simulink model "P4p3"  (R2014a)
settings: Solver=ode1  StartTime=0.0  StopTime=inf  FixedStep=0.002  RelTol=1e-3
PostLoadFcn:
  | qc_set_target_type(getConfigSet(bdroot, 'QUARC Default Target Configuration'));
undefined symbols (not defined in the file): A, B, C_elev_trav, HIL, Joystick_gain_x, Joystick_gain_y, K_P, L_elev_trav_real, P_P, qc_get_step_size, Vd_star, Vs_star
libraries: simulink_extras x6, quarc_library x4
settings Model: SimulationMode=external  ExtModeTrigDuration=15000  Creator=Rchan  LastModifiedBy=tikjetsa
settings SolverCC: PositivePriorityOrder=on
settings DataIOCC: SignalLoggingSaveFormat=ModelDataLogs
settings OptimizationCC: ExpressionDepthLimit=2147483647  InitFltsAndDblsToZero=on
settings DebuggingCC: SaveWithParameterizedLinksMsg=none  UnderspecifiedInitializationDetection=Classic  MultiTaskDSMMsg=warning  MultiTaskCondExecSysMsg=none  FcnCallInpInsideContextMsg=UseLocalSettings  StateNameClashWarn=warning
settings RTWCC: SystemTargetFile=quarc_win64.tlc  TemplateMakefile=quarc_default_tmf  Description=QUARC Win64 Target  ProcessScript=quarc_win64_make_rtw_hook
settings STFCustomTargetCC: CPPClassGenCompliant=on
settings GRTTargetCC: ParMdlRefBuildCompliant=off  CompOptLevelCompliant=off  CombineOutputUpdateFcns=off  MatFileLogging=off  GRTInterface=on  ExtMode=on  ExtModeMexFile=quarc_comm

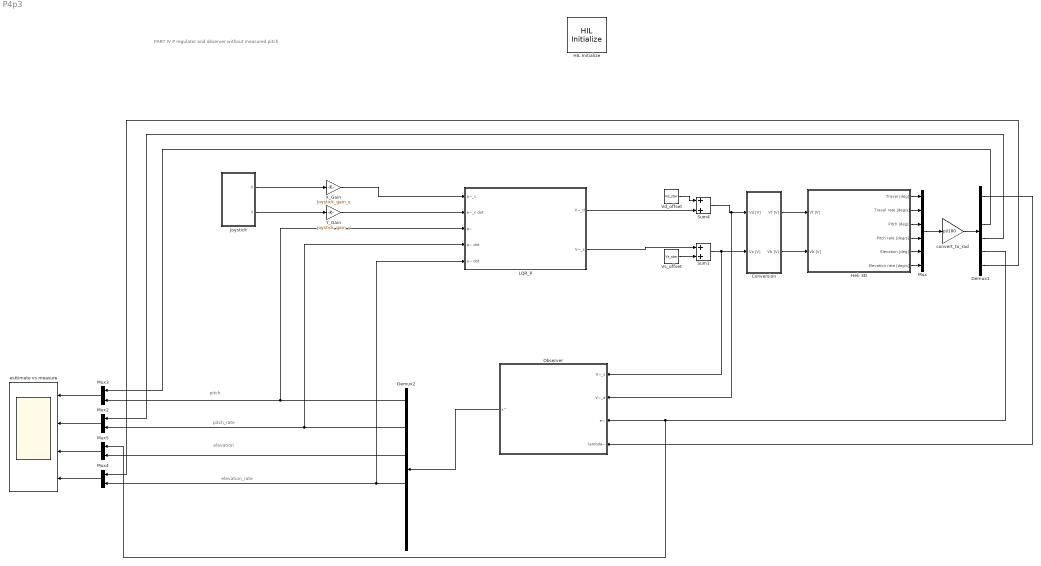
== system P4p3 ==
  note: elevation_rate
  note: elevation
  note: pitch_rate
  note: pitch
  note: PART IV
      | P regulator and observer without measured pitch
  Conversion : Subsystem
  Demux1 : Demux  Outputs=6
  Demux2 : Demux  Outputs=6
  HIL Initialize : quarc_library/Data Acquisition/Generic/Configuration/HIL Initialize  Priority=-99  object_name=HIL-1  board_type=q8_usb  board_number=0  board_options=update_rate=normal;decimation=1  exclusive=off  active=off  hardware_clocks=[0:2]  clock_modes=[]  initial_clock_frequencies=[]  set_clock_params_at_start=off  set_clock_params_at_switch_in=off  set_clock_frequencies_at_start=off  set_clock_frequencies_at_switch_in=off  analog_input_channels=[0:7]  analog_input_maximums=10  analog_input_minimums=-10  set_analog_input_params_at_start=on  set_analog_input_params_at_switch_in=off  analog_output_channels=[0:7]  analog_output_maximums=10  analog_output_minimums=-10  initial_analog_outputs=[0]  final_analog_outputs=[0]  watchdog_analog_outputs=0  set_analog_output_params_at_start=on  set_analog_output_params_at_switch_in=off  set_analog_outputs_at_start=on  set_analog_outputs_at_switch_in=off  set_analog_outputs_at_terminate=on  set_analog_outputs_at_switch_out=off  set_analog_outputs_on_watchdog=off  digital_input_channels=[]  digital_output_channels=[]  digital_output_configuration=[]  initial_digital_outputs=[1]  final_digital_outputs=[1]  watchdog_digital_outputs=[1]  set_digital_output_params_at_start=off  set_digital_output_params_at_switch_in=off  set_digital_outputs_at_start=on  set_digital_outputs_at_switch_in=off  set_digital_outputs_at_terminate=on  set_digital_outputs_at_switch_out=off  set_digital_outputs_on_watchdog=off  encoder_channels=[0:7]  quadrature=[4]  encoder_filter_frequency=[]  initial_encoder_counts=[0]  set_encoder_params_at_start=on  set_encoder_params_at_switch_in=off  set_encoder_counts_at_start=on  set_encoder_counts_at_switch_in=off  pwm_channels=[0:7]  pwm_modes=0  pwm_frequency=99.532799999999995e6/4095  pwm_configuration=[0]  pwm_alignment=[0]  pwm_polarity=[1]  pwm_leading_deadband=[0]  pwm_trailing_deadband=[0]  initial_pwm_outputs=[0]  final_pwm_outputs=[0]  watchdog_pwm_outputs=[0]  set_pwm_params_at_start=on  set_pwm_params_at_switch_in=off  set_pwm_outputs_at_start=on  set_pwm_outputs_at_switch_in=off  set_pwm_outputs_at_terminate=on  set_pwm_outputs_at_switch_out=off  set_pwm_outputs_on_watchdog=off  other_output_channels=[]  initial_other_outputs=[]  final_other_outputs=[]  watchdog_other_outputs=[]  set_other_outputs_at_start=off  set_other_outputs_at_switch_in=off  set_other_outputs_at_terminate=off  set_other_outputs_at_switch_out=off  set_other_outputs_on_watchdog=off
  Heli 3D : Subsystem
  Joystick : Subsystem
  LQR_P : Subsystem
  Mux : Mux  Inputs=6
  Mux{2..5} (4 alike) : Mux  Inputs=2
  Observer : Subsystem
  Sum1 : Sum
  Sum4 : Sum
  Vd_offset : Constant  Value=Vd_star
  Vs_offset : Constant  Value=Vs_star
  X_Gain : Gain  Gain=Joystick_gain_x
  Y_Gain : Gain  Gain=Joystick_gain_y
  convert_to_rad : Gain  Gain=pi/180
  esttimate vs measure : Scope  NumInputPorts=4
      settings: ShowLegends=on  YMin=-0.9~-1~0.48~-0.2  YMax=1~1.25~0.575~0.2  SaveName=ScopeData3
  wires:
  Conversion/2(Vb [V]) -> Heli 3D/2(Vb [V])
  Conversion/1(Vf [V]) -> Heli 3D/1(Vf [V])
  Heli 3D/1(Travel [deg]) -> Mux/1
  Heli 3D/2(Travel rate [deg/s]) -> Mux/2
  Heli 3D/3(Pitch [deg]) -> Mux/3
  Heli 3D/4(Pitch rate [deg/s]) -> Mux/4
  Heli 3D/5(Elevation [deg]) -> Mux/5
  Heli 3D/6(Elevation rate [deg/s]) -> Mux/6
  Mux/1 -> convert_to_rad/1
  convert_to_rad/1 -> Demux1/1
  Joystick/1(X) -> X_Gain/1
  Y_Gain/1 -> LQR_P/2(e~_c dot)
  Joystick/2(Y) -> Y_Gain/1
  X_Gain/1 -> LQR_P/1(p~_c)
  Sum4/1 -> Observer/2(V~_d), Conversion/1(Vd [V])
  Vd_offset/1 -> Sum4/1
  LQR_P/1(V~_d) -> Sum4/2
  Vs_offset/1 -> Sum1/2
  LQR_P/2(V~_s) -> Sum1/1
  Sum1/1 -> Observer/1(V~_s), Conversion/2(Vs [V])
  Demux1/1 -> Observer/4(lambda~)
  Demux1/5 -> Mux5/1, Observer/3(e~)
  Demux1/3 -> Mux3/1
  Demux1/4 -> Mux2/1
  Demux1/6 -> Mux4/1
  Observer/1(x^) -> Demux2/1
  Mux3/1 -> esttimate vs measure/1
  Mux2/1 -> esttimate vs measure/2
  Mux5/1 -> esttimate vs measure/3
  Mux4/1 -> esttimate vs measure/4
  Demux2/2 -> LQR_P/4(p~ dot), Mux2/2
  Demux2/3 -> Mux5/2
  Demux2/4 -> LQR_P/5(e~ dot), Mux4/2
  Demux2/1 -> LQR_P/3(p~), Mux3/2

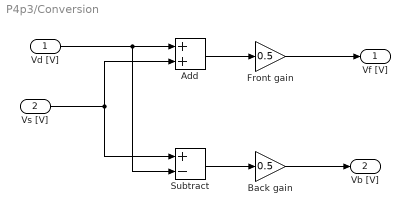
== system P4p3/Conversion ==
  Vd [V] : Inport
  Vs [V] : Inport  Port=2
  Add : Sum
  Back gain : Gain  Gain=0.5
  Front gain : Gain  Gain=0.5
  Subtract : Sum  Inputs=+-
  Vf [V] : Outport
  Vb [V] : Outport  Port=2
  wires:
  Vd [V]/1 -> Subtract/2, Add/1
  Vs [V]/1 -> Subtract/1, Add/2
  Subtract/1 -> Back gain/1
  Back gain/1 -> Vb [V]/1
  Add/1 -> Front gain/1
  Front gain/1 -> Vf [V]/1

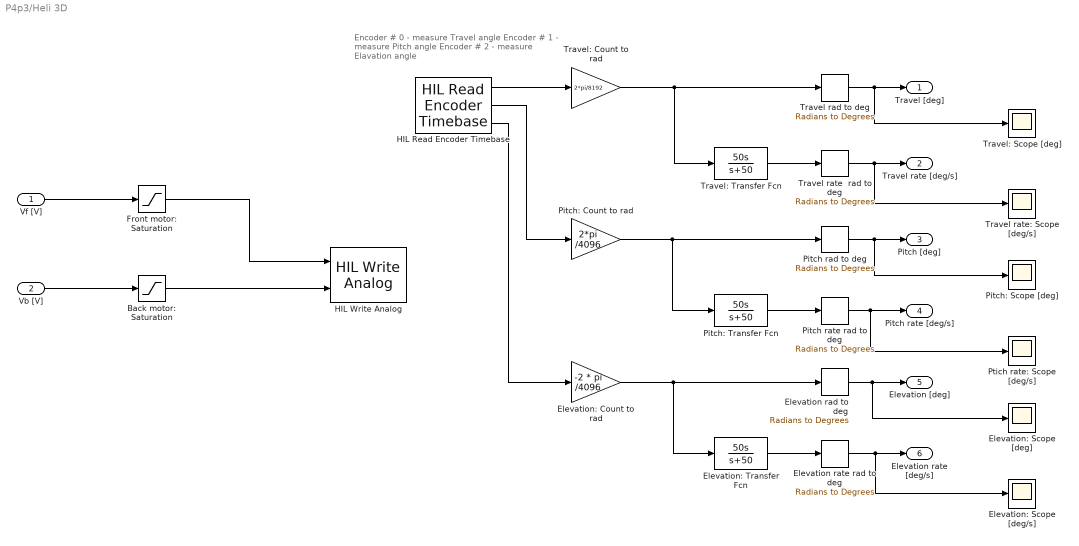
== system P4p3/Heli 3D ==
  note: Encoder # 0 - measure Travel angle
      | Encoder # 1 - measure Pitch angle
      | Encoder # 2 - measure Elavation angle
  Vf [V] : Inport
  Vb [V] : Inport  Port=2
  Back motor: Saturation : Saturate  UpperLimit=5  LowerLimit=-5
  Elevation rad to deg : simulink_extras/Transformations/Radians to Degrees
  Elevation rate rad to deg : simulink_extras/Transformations/Radians to Degrees
  Elevation: Count to rad : Gain  Gain=-2 * pi /4096
  Elevation: Scope [deg/s] : Scope
      settings: YMin=-15  YMax=15  SaveName=ScopeData13
  Elevation: Scope [deg] : Scope
      settings: YMin=-15  YMax=15  SaveName=ScopeData12
  Elevation: Transfer Fcn : TransferFcn  Numerator=[50 0]  Denominator=[1 50]
  Front motor: Saturation : Saturate  UpperLimit=5  LowerLimit=-5
  HIL Read Encoder Timebase : quarc_library/Data Acquisition/Generic/Timebases/HIL Read Encoder Timebase  object_name=HIL-1  clock=0  channels=[0:2]  samples_in_buffer=max(ceil(1/qc_get_step_size), 1)  active=on  vector_output=off  data_type_mode=Inherit via back propagation  data_type=double
  HIL Write Analog : quarc_library/Data Acquisition/Generic/Immediate I//O/HIL Write Analog  object_name=HIL-1  channels=[0:1]  sample_time=-1  active=off  vector_input=off
  Pitch rad to deg : simulink_extras/Transformations/Radians to Degrees
  Pitch rate rad to deg : simulink_extras/Transformations/Radians to Degrees
  Pitch: Count to rad : Gain  Gain=2*pi /4096
  Pitch: Scope [deg] : Scope
      settings: YMin=-15  YMax=15  SaveName=ScopeData10
  Pitch: Transfer Fcn : TransferFcn  Numerator=[50 0]  Denominator=[1 50]
  Ptich rate: Scope [deg/s] : Scope
      settings: YMin=-15  YMax=15  SaveName=ScopeData11
  Travel rad to deg : simulink_extras/Transformations/Radians to Degrees
  Travel rate  rad to deg : simulink_extras/Transformations/Radians to Degrees
  Travel rate: Scope [deg/s] : Scope
      settings: YMin=-15  YMax=15  SaveName=ScopeData9
  Travel: Count to rad : Gain  Gain=2*pi/8192
  Travel: Scope [deg] : Scope
      settings: YMin=-15  YMax=15  SaveName=ScopeData8
  Travel: Transfer Fcn : TransferFcn  Numerator=[50 0]  Denominator=[1 50]
  Travel [deg] : Outport
  Travel rate [deg/s] : Outport  Port=2
  Pitch [deg] : Outport  Port=3
  Pitch rate [deg/s] : Outport  Port=4
  Elevation [deg] : Outport  Port=5
  Elevation rate [deg/s] : Outport  Port=6
  wires:
  HIL Read Encoder Timebase/1 -> Travel: Count to rad/1
  HIL Read Encoder Timebase/2 -> Pitch: Count to rad/1
  HIL Read Encoder Timebase/3 -> Elevation: Count to rad/1
  Travel: Count to rad/1 -> Travel: Transfer Fcn/1, Travel rad to deg/1
  Travel: Transfer Fcn/1 -> Travel rate  rad to deg/1
  Pitch: Count to rad/1 -> Pitch: Transfer Fcn/1, Pitch rad to deg/1
  Pitch: Transfer Fcn/1 -> Pitch rate rad to deg/1
  Elevation: Count to rad/1 -> Elevation: Transfer Fcn/1, Elevation rad to deg/1
  Elevation: Transfer Fcn/1 -> Elevation rate rad to deg/1
  Travel rad to deg/1 -> Travel: Scope [deg]/1, Travel [deg]/1
  Travel rate  rad to deg/1 -> Travel rate: Scope [deg/s]/1, Travel rate [deg/s]/1
  Pitch rad to deg/1 -> Pitch: Scope [deg]/1, Pitch [deg]/1
  Pitch rate rad to deg/1 -> Ptich rate: Scope [deg/s]/1, Pitch rate [deg/s]/1
  Elevation rad to deg/1 -> Elevation: Scope [deg]/1, Elevation [deg]/1
  Elevation rate rad to deg/1 -> Elevation: Scope [deg/s]/1, Elevation rate [deg/s]/1
  Vf [V]/1 -> Front motor: Saturation/1
  Vb [V]/1 -> Back motor: Saturation/1
  Front motor: Saturation/1 -> HIL Write Analog/1
  Back motor: Saturation/1 -> HIL Write Analog/2

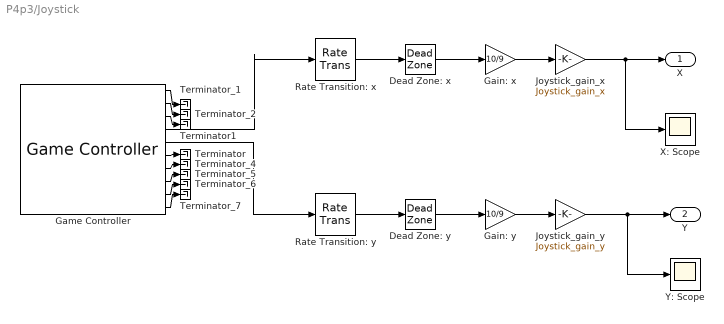
== system P4p3/Joystick ==
  Dead Zone: x : DeadZone  LowerValue=-0.1  UpperValue=0.1  SaturateOnIntegerOverflow=on
  Dead Zone: y : DeadZone  LowerValue=-0.1  UpperValue=0.1  SaturateOnIntegerOverflow=on
  Gain: x : Gain  Gain=10/9
  Gain: y : Gain  Gain=10/9
  Game Controller : quarc_library/Devices/Peripherals/Target/Game Controller  controller=1  buffer_size=12  deadzone=[]  saturation=[]  sample_time=max(qc_get_step_size, 0.01)  auto_center=off  enabled=on
  Joystick_gain_x : Gain  Gain=Joystick_gain_x
  Joystick_gain_y : Gain  Gain=Joystick_gain_y
  Rate Transition: x : RateTransition
  Rate Transition: y : RateTransition
  Terminator : Terminator
  Terminator1 : Terminator
  Terminator_{1..2,4..7} (6 alike) : Terminator
  X: Scope : Scope
      settings: YMin=-1  YMax=1  SaveName=ScopeData7
  Y: Scope : Scope
      settings: YMin=-10  YMax=10  SaveName=ScopeData5
  X : Outport
  Y : Outport  Port=2
  wires:
  Rate Transition: y/1 -> Dead Zone: y/1
  Rate Transition: x/1 -> Dead Zone: x/1
  Game Controller/5 -> Rate Transition: y/1
  Game Controller/4 -> Rate Transition: x/1
  Game Controller/1 -> Terminator_1/1
  Game Controller/2 -> Terminator_2/1
  Game Controller/7 -> Terminator_4/1
  Game Controller/8 -> Terminator_5/1
  Game Controller/9 -> Terminator_6/1
  Game Controller/10 -> Terminator_7/1
  Game Controller/3 -> Terminator1/1
  Game Controller/6 -> Terminator/1
  Dead Zone: x/1 -> Gain: x/1
  Dead Zone: y/1 -> Gain: y/1
  Gain: x/1 -> Joystick_gain_x/1
  Gain: y/1 -> Joystick_gain_y/1
  Joystick_gain_x/1 -> X/1, X: Scope/1
  Joystick_gain_y/1 -> Y: Scope/1, Y/1

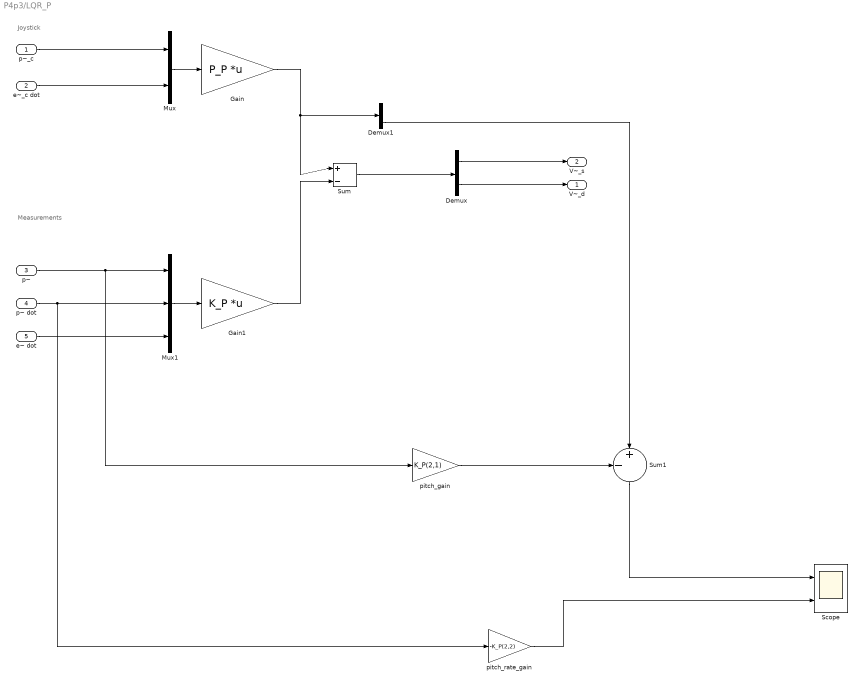
== system P4p3/LQR_P ==
  note: Joystick
  note: Measurements
  p~_c : Inport
  e~_c dot : Inport  Port=2
  p~ : Inport  Port=3
  p~ dot : Inport  Port=4
  e~ dot : Inport  Port=5
  Demux : Demux  Outputs=2
  Demux1 : Demux  Outputs=2
  Gain : Gain  Gain=P_P  Multiplication=Matrix(K*u) (u vector)
  Gain1 : Gain  Gain=K_P  Multiplication=Matrix(K*u) (u vector)
  Mux : Mux  Inputs=2
  Mux1 : Mux  Inputs=3
  Scope : Scope  NumInputPorts=2
      settings: ShowLegends=on  YMin=-10~-10  YMax=10~10  SaveName=ScopeData4
  Sum : Sum  Inputs=|+-
  Sum1 : Sum  Inputs=-+|
  pitch_gain : Gain  Gain=K_P(2,1)
  pitch_rate_gain : Gain  Gain=-K_P(2,2)
  V~_d : Outport
  V~_s : Outport  Port=2
  wires:
  p~_c/1 -> Mux/1
  e~_c dot/1 -> Mux/2
  Mux/1 -> Gain/1
  Gain/1 -> Demux1/1, Sum/1
  Mux1/1 -> Gain1/1
  e~ dot/1 -> Mux1/3
  Gain1/1 -> Sum/2
  Sum/1 -> Demux/1
  Demux/1 -> V~_s/1
  Demux/2 -> V~_d/1
  p~/1 -> pitch_gain/1, Mux1/1
  p~ dot/1 -> pitch_rate_gain/1, Mux1/2
  pitch_rate_gain/1 -> Scope/2
  Demux1/2 -> Sum1/2
  pitch_gain/1 -> Sum1/1
  Sum1/1 -> Scope/1

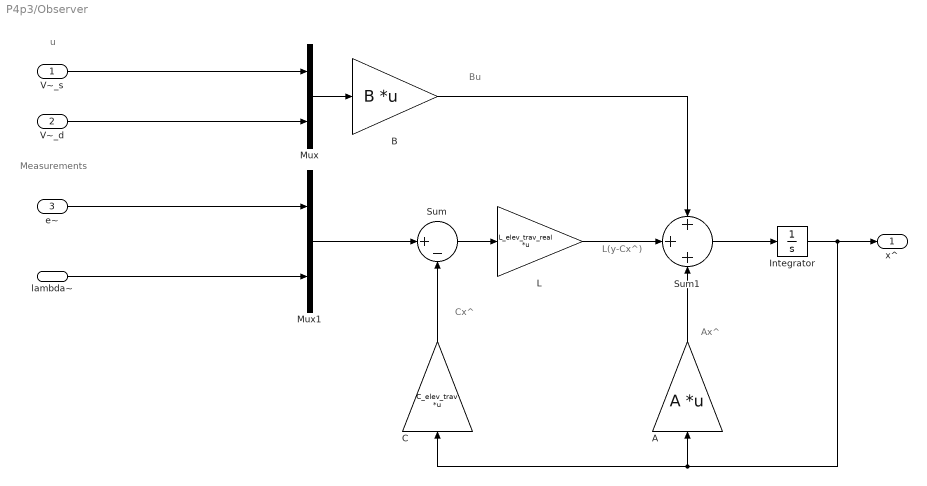
== system P4p3/Observer ==
  note: L(y-Cx^)
  note: Cx^
  note: Ax^
  note: Bu
  note: Measurements
  note: u
  V~_s : Inport
  V~_d : Inport  Port=2
  e~ : Inport  Port=3
  lambda~ : Inport  Port=4
  A : Gain  Gain=A  Multiplication=Matrix(K*u) (u vector)
  B : Gain  Gain=B  Multiplication=Matrix(K*u) (u vector)
  C : Gain  Gain=C_elev_trav  Multiplication=Matrix(K*u) (u vector)
  Integrator : Integrator
  L : Gain  Gain=L_elev_trav_real  Multiplication=Matrix(K*u) (u vector)
  Mux : Mux  Inputs=2
  Mux1 : Mux  Inputs=2
  Sum : Sum  Inputs=|+-
  Sum1 : Sum  Inputs=+++
  x^ : Outport
  wires:
  V~_s/1 -> Mux/1
  V~_d/1 -> Mux/2
  Mux/1 -> B/1
  e~/1 -> Mux1/1
  lambda~/1 -> Mux1/2
  Sum/1 -> L/1
  L/1 -> Sum1/2
  B/1 -> Sum1/1
  Sum1/1 -> Integrator/1
  Mux1/1 -> Sum/1
  Integrator/1 -> C/1, A/1, x^/1
  A/1 -> Sum1/3
  C/1 -> Sum/2
